simulink model "time_to_zero_vertical_velocity"  (R2020b)
settings: Solver=FixedStepAuto  StartTime=0.0  StopTime=10.0  RelTol=1e-3
settings Model: Creator=wizard  LastModifiedBy=Nicolai

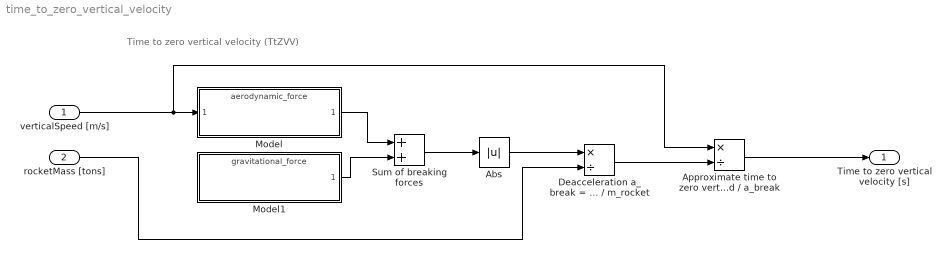
== system time_to_zero_vertical_velocity ==
  note: Time to zero vertical velocity (TtZVV)
  verticalSpeed [m/s] : Inport
  rocketMass [tons] : Inport  Port=2
  Abs : Abs
  Approximate time to zero vertical velocity t_zvv = verticalSpeed / a_break : Product  Inputs=*/
  Deacceleration a_break = F_break / m_rocket : Product  Inputs=*/
  Model : ModelReference  ModelNameDialog=aerodynamic_force.slx  SimulationMode=Normal  ModelReferenceVersion=1.5
  Model1 : ModelReference  ModelNameDialog=gravitational_force.slx  SimulationMode=Normal  ModelReferenceVersion=1.4
  Sum of breaking forces : Sum
  Time to zero vertical velocity [s] : Outport
  wires:
  Abs/1 -> Deacceleration a_break = F_break / m_rocket/1
  Approximate time to zero vertical velocity t_zvv = verticalSpeed / a_break/1 -> Time to zero vertical velocity [s]/1
  Sum of breaking forces/1 -> Abs/1
  verticalSpeed [m/s]/1 -> Approximate time to zero vertical velocity t_zvv = verticalSpeed / a_break/1, Model/1
  Model/1 -> Sum of breaking forces/1
  Deacceleration a_break = F_break / m_rocket/1 -> Approximate time to zero vertical velocity t_zvv = verticalSpeed / a_break/2
  rocketMass [tons]/1 -> Deacceleration a_break = F_break / m_rocket/2
  Model1/1 -> Sum of breaking forces/2
